simulink model "house_heat_model"  (R2017a)
settings: Solver=ode3  StartTime=0.0  StopTime=1*7*24*3600  FixedStep=dt  RelTol=1e-3  AbsTol=1e-6
model workspace (MATLAB code in the model file):
  | % load initial conditions and physical properties from file
  | 
  | house_heat_model_init
values from neighbouring files (symbols this model uses):
  c_a = simdata.Simulation.Material.c_a.value    [house_heat_model_init.m]
  c_floor = simdata.Simulation.Material.c_floor.value    [house_heat_model_init.m]
  c_s = simdata.Simulation.Material.c_s.value    [house_heat_model_init.m]
  c_water = simdata.Simulation.Material.c_water.value    [house_heat_model_init.m]
  dt = simdata.Simulation.dt.value    [house_heat_model_init.m]
  dT_histerezis = simdata.Simulation.Heat.dT_histerizes.value    [house_heat_model_init.m]
  M_air = (lenHouse*widHouse*htHouse+tan(pitRoof)*widHouse*lenHouse)*densAir    [house_heat_model_init.m]
  M_floor = floorArea*L_floor*densConcrete*heatedPct    [house_heat_model_init.m]
  Mdot = simdata.Simulation.Heat.M_dot.value    [house_heat_model_init.m]
  R_floor = L_floor/(k_floor*floorArea)    [house_heat_model_init.m]
  R_house = R_wall*R_window/(R_wall + R_window)    [house_heat_model_init.m]
  THeater = simdata.Simulation.Heat.T_Heater.value    [house_heat_model_init.m]
  TinIC = simdata.Simulation.Heat.T_IN_ini.value    [house_heat_model_init.m]
libraries: neural x15, dspswit3 x1, simulink x1, powerlib_meascontrol x1
settings Model: ExtModeTrigMode=oneshot  ExtModeArmWhenConnect=off  ExtModeAutoUpdateStatusClock=off  Creator=The MathWorks Inc.  LastModifiedBy=szabo
settings DataIOCC: Decimation=5  ExternalInput=[]  InitialState=[]  SaveFormat=Array  SaveOutput=off  SignalLogging=off  SaveTime=off  SignalLoggingName=sldemo_househeat_output
settings OptimizationCC: BlockReduction=off  BooleanDataType=off  ExpressionDepthLimit=2147483647  InitFltsAndDblsToZero=on  LifeSpan=inf  BufferReusableBoundary=off
settings DebuggingCC: SaveWithParameterizedLinksMsg=none  UnderspecifiedInitializationDetection=Classic  MergeDetectMultiDrivingBlocksExec=none  SignalResolutionControl=TryResolveAllWithWarning  MultiTaskDSMMsg=warning  MultiTaskCondExecSysMsg=none  IntegerOverflowMsg=none  FcnCallInpInsideContextMsg=warning  BusObjectLabelMismatch=none  StateNameClashWarn=warning  SFUnexpectedBacktrackingDiag=warning  SFNoUnconditionalDefaultTransitionDiag=warning  SFExecutionAtInitializationDiag=none  IntegerSaturationMsg=none
settings HardwareCC: ProdBitPerPointer=32  ProdBitPerSizeT=32  ProdBitPerPtrDiffT=32  ProdLargestAtomicFloat=None  ProdIntDivRoundTo=Undefined  ProdEndianess=Unspecified  ProdWordSize=32  ProdHWDeviceType=32-bit Generic  TargetUnknown=on
settings ModelReferenceCC: PropagateSignalLabelsOutOfModel=off
settings GRTTargetCC: TargetFcnLib=ansi_tfl_tmw.mat  TargetLangStandard=C89/C90 (ANSI)  GeneratePreprocessorConditionals=Disable all  CombineOutputUpdateFcns=off  GRTInterface=on
settings ConfigComp: CovMetricSettings=dw  CovHtmlReporting=on  CovSaveCumulativeToWorkspaceVar=on  CovSaveSingleToWorkspaceVar=on  CovExternalEMLEnable=off  CovSFcnEnable=off

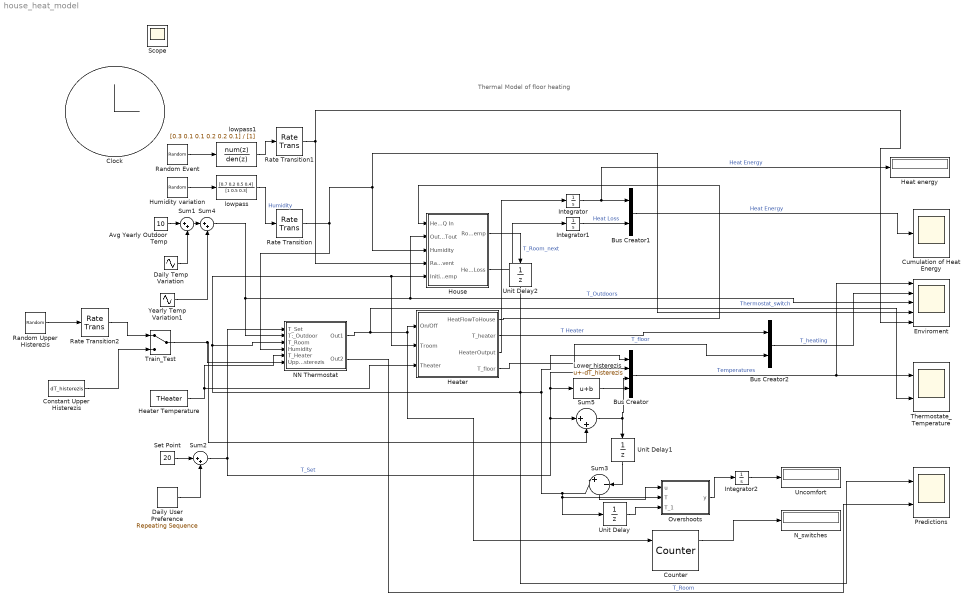
== system house_heat_model ==
  note: Thermal Model of floor heating
  Avg Yearly Outdoor Temp : Constant  Value=10
  Bus Creator : BusCreator  Inputs=4
  Bus Creator1 : BusCreator  Inputs=2
  Bus Creator2 : BusCreator  Inputs=2
  Clock : Clock
  Constant Upper Histerezis : Constant  Value=dT_histerezis  SampleTime=dt
  Counter : dspswit3/Counter  Direction=Up  CountEvent=Rising edge  CounterSize=32 bits  MaxCount=255  InitialCount=0  Output=Count and Hit  HitValue=32  ResetInput=on  SamplesPerFrame=1  Ts=1  CntDtype=double  HitDtype=Logical
  Cumulation of Heat Energy : Scope
  Daily Temp Variation : Sin  Amplitude=5  Frequency=2*pi/(24*3600)  SampleTime=dt
  Daily User Preference : simulink/Sources/Repeating Sequence  rep_seq_t=[0 25199 25200 32399 32400 57599 57600 79199 79200]  rep_seq_y=[-1 -1 1 1 -2 -2 1 1 -1]
  Enviroment : Scope  NumInputPorts=5
  Heat energy : Display
  Heater : Subsystem
      settings: MinAlgLoopOccurrences=on
  Heater Temperature : Constant  Value=THeater
  House : Subsystem
      settings: MinAlgLoopOccurrences=on
      mask Display: image(fullfile(matlabroot,'toolbox','simulink','simdemos','simgeneral','images','HouseHeatHousePix.svg'))
  Humidity variation : RandomNumber  Description=Random events in heat capacity of the room - like window opening, persons in the house, e.t.c  Mean=0.7  Variance=0.05  SampleTime=3600*24
  Integrator : Integrator
  Integrator1 : Integrator
  Integrator2 : Integrator
  Lower histerezis : Bias  Bias=-dT_histerezis
  "NN Thermostat " : Subsystem
      settings: MinAlgLoopOccurrences=on
      mask Display: image(fullfile(matlabroot,'toolbox','simulink','simdemos','simgeneral','images','HouseHeatThermostatPix.svg'))
  N_switches : Display
  Overshoots : MATLAB Function  TreatAsAtomicUnit=on
  Predictions : Scope  NumInputPorts=2
  Random Event : RandomNumber  Mean=1.2  Variance=0.01  SampleTime=3600
  Random Upper Histerezis : UniformRandomNumber  Minimum=0  Maximum=dT_histerezis  SampleTime=3600
  Rate Transition : RateTransition  X0=0.7
  Rate Transition1 : RateTransition  X0=1
  Rate Transition2 : RateTransition  X0=0.25
  Set Point : Constant  Value=20
  Sum{1..2,4..5} (4 alike) : Sum  Inputs=|++  SaturateOnIntegerOverflow=on  InputSameDT=on  OutDataTypeStr=Inherit: Same as first input
  Sum3 : Sum  Inputs=|+||-  SaturateOnIntegerOverflow=on  InputSameDT=on  OutDataTypeStr=Inherit: Same as first input
  Thermostate_Temperature : Scope  NumInputPorts=2
  Train_Test : ManualSwitch
  Uncomfort : Display
  Unit Delay : UnitDelay  InitialCondition=TinIC  SampleTime=-1
  Unit Delay1 : UnitDelay  InitialCondition=TinIC  SampleTime=-1
  Unit Delay2 : UnitDelay  InitialCondition=TinIC  SampleTime=-1
  Yearly Temp Variation1 : Sin  Amplitude=10  Frequency=2*pi/(365*24*3600)  Phase=-3*pi/4  SampleTime=dt
  lowpass : DiscreteFilter  Numerator=[0.7 0.2 0.5 0.4]  Denominator=[1 0.5 0.3]  InitialStates=0.5  SampleTime=3600  a0EqualsOne=on
  lowpass1 : DiscreteFilter  Numerator=[0.3 0.1 0.1 0.2 0.2 0.1]  Denominator=[1]  InitialStates=1  SampleTime=120  a0EqualsOne=on
  Scope : Scope
  wires:
  Integrator/1 -> Heat energy/1, Bus Creator1/1  "Heat Energy"
  Daily Temp Variation/1 -> Sum1/2
  Sum4/1 -> "NN Thermostat "/2(T:_Outdoor), Enviroment/3, House/2(Outdoor Temp Tout)  "T_Outdoors"
  Avg Yearly Outdoor Temp/1 -> Sum1/1
  House/1("Room Temp ") -> Unit Delay2/1  "T_Room_next"
  Heater/1("HeatFlowToHouse ") -> House/1(Heater dQ In)
  Daily User Preference/1 -> Sum2/2
  Set Point/1 -> Sum2/1
  Sum2/1 -> "NN Thermostat "/1(T_Set), Sum5/1, Lower histerezis/1, Bus Creator/2  "T_Set"
  Bus Creator/1 -> Enviroment/1, Thermostate_Temperature/1  "Temperatures"
  Sum5/1 -> Bus Creator/3, Unit Delay1/1
  Random Event/1 -> lowpass1/1
  Heater/3(HeaterOutput) -> Integrator/1
  House/2(Heat Loss) -> Integrator1/1
  Integrator1/1 -> Bus Creator1/2  "Heat Loss"
  Overshoots/1(y) -> Integrator2/1
  Integrator2/1 -> Uncomfort/1
  Counter/1 -> N_switches/1
  Humidity variation/1 -> lowpass/1
  lowpass/1 -> Rate Transition/1  "Humidity"
  lowpass1/1 -> Rate Transition1/1
  "NN Thermostat "/1(Out1) -> Thermostate_Temperature/2, Counter/1, Heater/1(On/Off)  "Thermostat_switch"
  Unit Delay2/1 -> Predictions/1, Heater/2(Troom), House/5("Initial Room Temp "), "NN Thermostat "/3(T_Room), Bus Creator/1, Sum3/1, Overshoots/2(T), Unit Delay/1  "T_Room"
  Sum3/1 -> Overshoots/1(u)
  Unit Delay/1 -> Overshoots/3(T_1)
  Unit Delay1/1 -> Sum3/2
  Lower histerezis/1 -> Bus Creator/4
  "NN Thermostat "/2(Out2) -> Predictions/2
  Rate Transition/1 -> House/3(Humidity), Enviroment/4, "NN Thermostat "/4(Humidity)
  Rate Transition1/1 -> House/4("Random Event "), Enviroment/5
  Heater Temperature/1 -> "NN Thermostat "/5(T_Heater), Heater/3(Theater)
  Sum1/1 -> Sum4/1
  Yearly Temp Variation1/1 -> Sum4/2
  Bus Creator2/1 -> Enviroment/2  "T_heatiing"
  Heater/2("T_heater ") -> Bus Creator2/1  "T Heater"
  Heater/4(T_floor) -> Bus Creator2/2  "T_floor"
  Random Upper Histerezis/1 -> Rate Transition2/1
  Train_Test/1 -> Sum5/2, "NN Thermostat "/6(Upper Histerezis)
  Constant Upper Histerezis/1 -> Train_Test/2
  Rate Transition2/1 -> Train_Test/1
  Bus Creator1/1 -> Cumulation of Heat Energy/1  "Heat Energy"

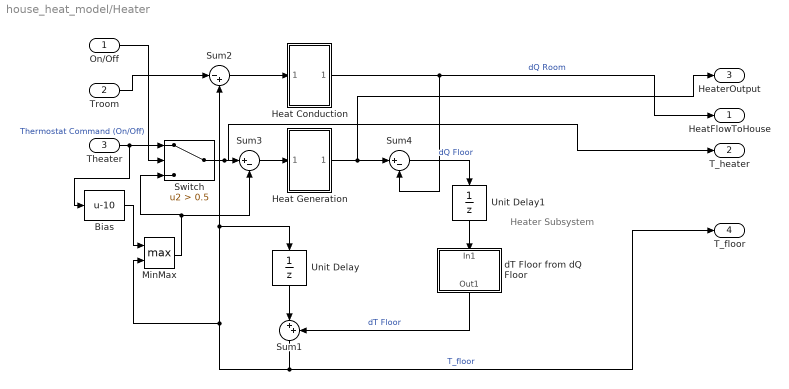
== system house_heat_model/Heater ==
  note: Heater Subsystem
  On/Off : Inport
  Troom : Inport  Port=2
  Theater : Inport  Port=3
  Bias : Bias  Bias=-10
  Heat Generation : Subsystem  Description=assumption: all heater energy is transmitted to the floor and house heating
  Heat Conduction : Subsystem
  MinMax : MinMax  Function=max  Inputs=2
  Sum1 : Sum  Inputs=|++
  Sum2 : Sum  Inputs=|-+
  Sum3 : Sum  Inputs=|+-
  Sum4 : Sum  Inputs=|+-
  Switch : Switch  Criteria=u2 > Threshold  Threshold=0.5
  Unit Delay : UnitDelay  InitialCondition=TinIC  SampleTime=-1
  Unit Delay1 : UnitDelay  InitialCondition=TinIC  SampleTime=-1
  dT Floor from dQ Floor : Subsystem
  "HeatFlowToHouse " : Outport
  "T_heater " : Outport  Port=2
  HeaterOutput : Outport  Port=3
  T_floor : Outport  Port=4
  wires:
  Troom/1 -> Sum2/1
  Sum2/1 -> Heat Conduction/1(In1)
  On/Off/1 -> Switch/2  "Thermostat Command (On/Off)"
  Unit Delay/1 -> Sum1/1
  Sum1/1 -> MinMax/2, Sum2/2, Unit Delay/1, T_floor/1  "T_floor"
  Theater/1 -> Bias/1, Switch/1
  dT Floor from dQ Floor/1(Out1) -> Sum1/2  "dT Floor"
  Heat Conduction/1(Out1) -> "HeatFlowToHouse "/1, Sum4/2  "dQ Room"
  Switch/1 -> "T_heater "/1, Sum3/1
  Sum3/1 -> Heat Generation/1(In1)
  Heat Generation/1(Out1) -> HeaterOutput/1, Sum4/1
  Sum4/1 -> Unit Delay1/1  "dQ Floor"
  Unit Delay1/1 -> dT Floor from dQ Floor/1(In1)
  Bias/1 -> MinMax/1
  MinMax/1 -> Sum3/2, Switch/3

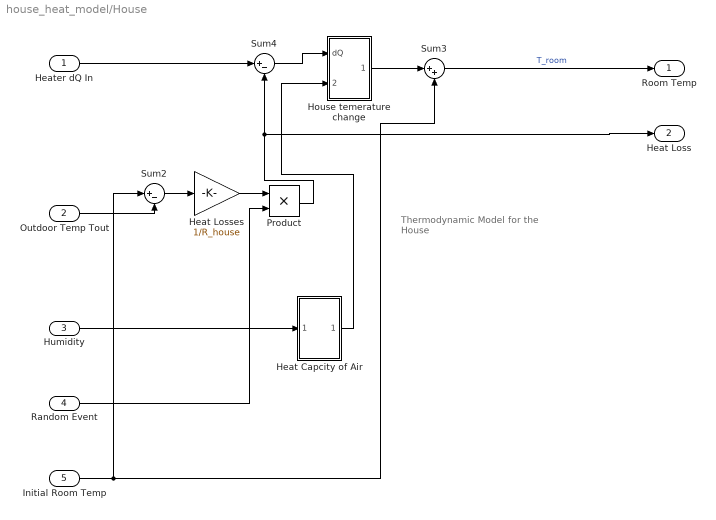
== system house_heat_model/House ==
  note: Thermodynamic Model
      | for the House
  Heater dQ In : Inport
  Outdoor Temp Tout : Inport  Port=2
  Humidity : Inport  Port=3
  "Random Event " : Inport  Port=4
  "Initial Room Temp " : Inport  Port=5
  "Heat Capcity of Air " : Subsystem
  Heat Losses : Gain  Gain=1/R_house  SaturateOnIntegerOverflow=on  OutDataTypeStr=Inherit: Same as input  ParamDataTypeStr=Inherit: Same as input
  House temerature change : Subsystem
  Product : Product
  Sum2 : Sum  Inputs=|+-  SaturateOnIntegerOverflow=on  InputSameDT=on  OutDataTypeStr=Inherit: Same as first input
  Sum3 : Sum  Inputs=|++
  Sum4 : Sum  Inputs=|+-  SaturateOnIntegerOverflow=on  InputSameDT=on  OutDataTypeStr=Inherit: Same as first input
  "Room Temp " : Outport  InitialOutput=0
  Heat Loss : Outport  Port=2  InitialOutput=0
  wires:
  Outdoor Temp Tout/1 -> Sum2/2
  Sum2/1 -> Heat Losses/1
  Sum3/1 -> "Room Temp "/1  "T_room"
  Heater dQ In/1 -> Sum4/1
  House temerature change/1(Out1) -> Sum3/1
  Sum4/1 -> House temerature change/1(dQ)
  Humidity/1 -> "Heat Capcity of Air "/1(In1)
  "Heat Capcity of Air "/1(Out1) -> House temerature change/2(Heat Capacity)
  "Random Event "/1 -> Product/2
  Heat Losses/1 -> Product/1
  Product/1 -> Heat Loss/1, Sum4/2
  "Initial Room Temp "/1 -> Sum2/1, Sum3/2

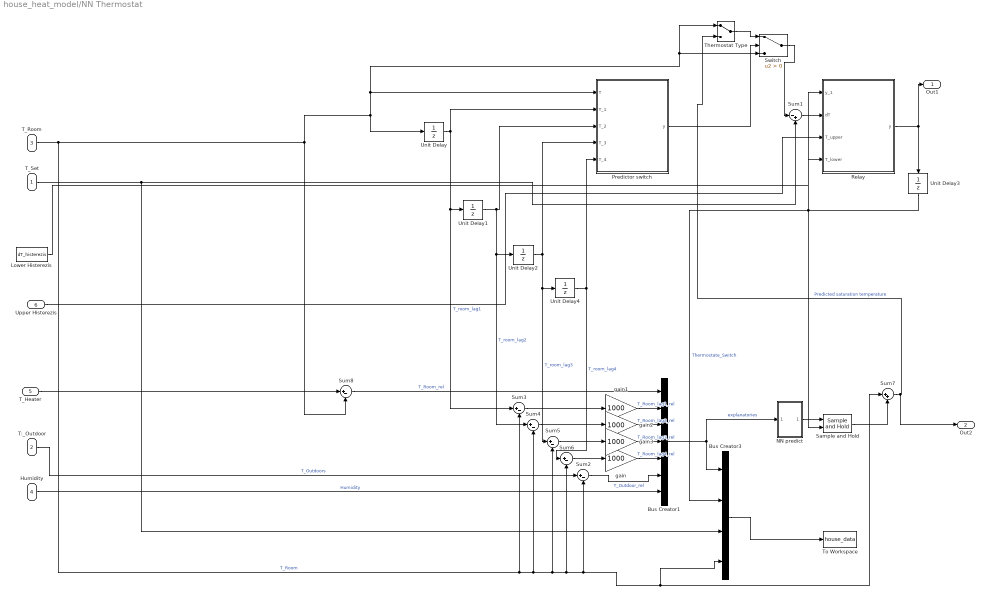
== system house_heat_model/NN Thermostat  ==
  T_Set : Inport
  T:_Outdoor : Inport  Port=2
  T_Room : Inport  Port=3
  Humidity : Inport  Port=4
  T_Heater : Inport  Port=5
  Upper Histerezis : Inport  Port=6
  Bus Creator1 : BusCreator  Inputs=7
  Bus Creator3 : BusCreator  Inputs=4
  Lower Histerezis : Constant  Value=dT_histerezis
  NN predict : Subsystem
  Predictor switch : MATLAB Function  TreatAsAtomicUnit=on
  Relay : MATLAB Function  TreatAsAtomicUnit=on
  Sample and Hold : powerlib_meascontrol/Additional Components/Sample and Hold  ic=0  Ts=dt
      settings: SourceProductName=Simscape Power Systems  SourceProductBaseCode=PS
  Sum1 : Sum  Inputs=|-+  SaturateOnIntegerOverflow=on  InputSameDT=on  OutDataTypeStr=Inherit: Same as first input
  Sum{2..6,8} (6 alike) : Sum  Inputs=|+-  SaturateOnIntegerOverflow=on  InputSameDT=on  OutDataTypeStr=Inherit: Same as first input
  Sum7 : Sum  Inputs=|++  SaturateOnIntegerOverflow=on  InputSameDT=on  OutDataTypeStr=Inherit: Same as first input
  Switch : Switch  Criteria=u2 > Threshold
  Thermostat Type : ManualSwitch  Description=|
      | Turn on/off smart thermostat
      | Off: Up
      | On: Down
  To Workspace : ToWorkspace  VariableName=house_data  SaveFormat=Timeseries  SampleTime=-1
  Unit Delay{,1..2,4} (4 alike) : UnitDelay  InitialCondition=TinIC  SampleTime=-1
  Unit Delay3 : UnitDelay  SampleTime=-1
  gain{,1..3} (4 alike) : Gain  Gain=1000
  Out1 : Outport
  Out2 : Outport  Port=2
  wires:
  Unit Delay/1 -> Predictor switch/2(T_1), Sum3/1, Unit Delay1/1  "T_room_lag1"
  Relay/1(y) -> Out1/1, Unit Delay3/1
  Switch/1 -> Sum1/1
  Unit Delay1/1 -> Predictor switch/3(T_2), Unit Delay2/1, Sum4/1  "T_room_lag2"
  Predictor switch/1(y) -> Switch/2
  Unit Delay2/1 -> Unit Delay4/1, Sum5/1, Predictor switch/4(T_3)  "T_room_lag3"
  Unit Delay3/1 -> Relay/1(y_1), Sample and Hold/2, Bus Creator3/2  "Thermostate_Switch"
  Thermostat Type/1 -> Switch/1
  T_Room/1 -> Sum8/2, Predictor switch/1(T), Thermostat Type/1, Switch/3, Unit Delay/1, Sum7/1, Bus Creator3/4, Sum2/2, Sum6/2, Sum5/2, Sum4/2, Sum3/2  "T_Room"
  Bus Creator3/1 -> To Workspace/1
  NN predict/1(Out1) -> Sample and Hold/1
  Sum3/1 -> gain1/1
  Sum4/1 -> gain2/1
  Sum5/1 -> gain3/1
  Sum6/1 -> gain/1
  Humidity/1 -> Bus Creator1/7  "Humidity"
  Bus Creator1/1 -> NN predict/1(In1), Bus Creator3/1  "explanatories"
  Sample and Hold/1 -> Sum7/2
  T_Set/1 -> Bus Creator3/3, Sum1/2
  Sum7/1 -> Out2/1, Thermostat Type/2  "Predicted saturation temperature"
  Sum2/1 -> Bus Creator1/6  "T_Outdoor_rel"
  Unit Delay4/1 -> Predictor switch/5(T_4), Sum6/1  "T_room_lag4"
  T:_Outdoor/1 -> Sum2/1  "T_Outdoors"
  T_Heater/1 -> Sum8/1
  Sum8/1 -> Bus Creator1/1  "T_Room_rel"
  Lower Histerezis/1 -> Relay/4(T_lower)
  Upper Histerezis/1 -> Relay/3(T_upper)
  gain1/1 -> Bus Creator1/2  "T_Room_lag1_rel"
  gain2/1 -> Bus Creator1/3  "T_Room_lag2_rel"
  gain3/1 -> Bus Creator1/4  "T_Room_lag3_rel"
  gain/1 -> Bus Creator1/5  "T_Room_lag4_rel"
  Sum1/1 -> Relay/2(dT)

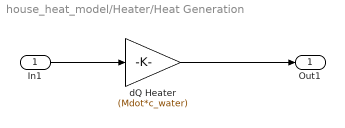
== system house_heat_model/Heater/Heat Generation ==
  In1 : Inport
  dQ Heater : Gain  Gain=(Mdot*c_water)
  Out1 : Outport
  wires:
  In1/1 -> dQ Heater/1
  dQ Heater/1 -> Out1/1

== system house_heat_model/Heater/Heat Conduction ==
  In1 : Inport
  Heat conduction : Gain  Gain=1/R_floor
  Out1 : Outport
  wires:
  In1/1 -> Heat conduction/1
  Heat conduction/1 -> Out1/1

== system house_heat_model/Heater/dT Floor from dQ Floor ==
  In1 : Inport
  Floor Incapacity : Gain  Gain=dt/(M_floor*c_floor)
  Out1 : Outport
  wires:
  In1/1 -> Floor Incapacity/1
  Floor Incapacity/1 -> Out1/1  "dT Floor"

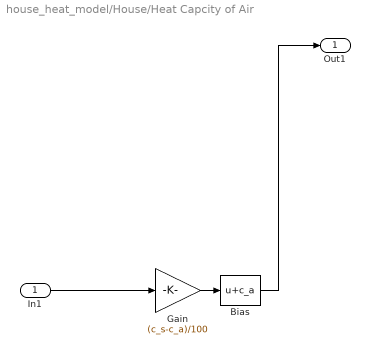
== system house_heat_model/House/Heat Capcity of Air  ==
  In1 : Inport
  Bias : Bias  Bias=c_a
  Gain : Gain  Gain=(c_s-c_a)/100  SaturateOnIntegerOverflow=on  OutDataTypeStr=Inherit: Same as input  ParamDataTypeStr=Inherit: Same as input
  Out1 : Outport
  wires:
  In1/1 -> Gain/1
  Bias/1 -> Out1/1
  Gain/1 -> Bias/1

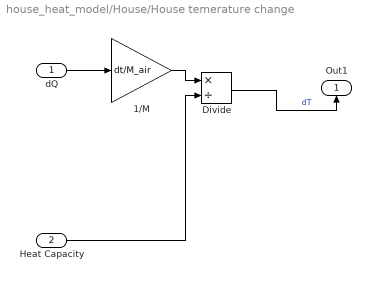
== system house_heat_model/House/House temerature change ==
  dQ : Inport
  Heat Capacity : Inport  Port=2
  1/M : Gain  Gain=dt/M_air  SaturateOnIntegerOverflow=on  OutDataTypeStr=Inherit: Same as input  ParamDataTypeStr=Inherit: Same as input
  Divide : Product  Inputs=*/
  Out1 : Outport
  wires:
  1/M/1 -> Divide/1
  dQ/1 -> 1/M/1
  Divide/1 -> Out1/1  "dT"
  Heat Capacity/1 -> Divide/2

== system house_heat_model/NN Thermostat /NN predict ==
  In1 : Inport
  Function Fitting Neural Network1 : Subsystem
      mask help: Function Fitting Neural Network
      mask Display: e = 0.06;c1 = [120 150 230]/255;c2 = ([120 150 230]+0)/383;c3 = ([120 150 230]+128)/383;patch([0 1 1 0],[0 0 1 1],c1);patch([0 1 1 1-e 1-e 0+e],[0 0 1 1-e 0+e 0+e],c2);patch([0 0 1 1-e 0+e 0+e],[0 1 1 1-e 1-e 0+e],c3);plot([0 1 1 0 0],[0 0 1 1 0]);fprintf('NNET');port_label('input',1,' Input');port_label('output',1,'Output ');
  Out1 : Outport
  wires:
  In1/1 -> Function Fitting Neural Network1/1(Input)
  Function Fitting Neural Network1/1(Output) -> Out1/1

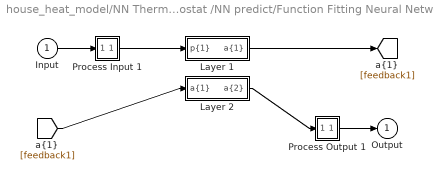
== system house_heat_model/NN Thermostat /NN predict/Function Fitting Neural Network1 ==
  Input : Inport  PortDimensions=7  SampleTime=10
      mask Display: e = 0.06;c1 = [120 230 180]/255;c2 = ([120 230 180]+0)/(256+128);c3 = ([120 230 180]+128)/(256+128);patch([0 1 1 0],[0 0 1 1],c1);patch([0 1 1 1-e 1-e 0+e],[0 0 1 1-e 0+e 0+e],c2);patch([0 0 1 1-e 0+e 0+e],[0 1 1 1-e 1-e 0+e],c3);plot([0 1 1 0 0],[0 0 1 1 0]);
  Layer 1 : Subsystem
      mask Display: e = 0.06;c1 = [120 150 230]/255;c2 = ([120 150 230]+0)/383;c3 = ([120 150 230]+128)/383;patch([0 1 1 0],[0 0 1 1],c1);patch([0 1 1 1-e 1-e 0+e],[0 0 1 1-e 0+e 0+e],c2);patch([0 0 1 1-e 0+e 0+e],[0 1 1 1-e 1-e 0+e],c3);plot([0 1 1 0 0],[0 0 1 1 0]);
  Layer 2 : Subsystem
      mask Display: e = 0.06;c1 = [120 150 230]/255;c2 = ([120 150 230]+0)/383;c3 = ([120 150 230]+128)/383;patch([0 1 1 0],[0 0 1 1],c1);patch([0 1 1 1-e 1-e 0+e],[0 0 1 1-e 0+e 0+e],c2);patch([0 0 1 1-e 0+e 0+e],[0 1 1 1-e 1-e 0+e],c3);plot([0 1 1 0 0],[0 0 1 1 0]);
  Process Input 1 : Subsystem
      mask Display: e = 0.06;c1 = [120 150 230]/255;c2 = ([120 150 230]+0)/383;c3 = ([120 150 230]+128)/383;patch([0 1 1 0],[0 0 1 1],c1);patch([0 1 1 1-e 1-e 0+e],[0 0 1 1-e 0+e 0+e],c2);patch([0 0 1 1-e 0+e 0+e],[0 1 1 1-e 1-e 0+e],c3);plot([0 1 1 0 0],[0 0 1 1 0]);
  Process Output 1 : Subsystem
      mask Display: e = 0.06;c1 = [120 150 230]/255;c2 = ([120 150 230]+0)/383;c3 = ([120 150 230]+128)/383;patch([0 1 1 0],[0 0 1 1],c1);patch([0 1 1 1-e 1-e 0+e],[0 0 1 1-e 0+e 0+e],c2);patch([0 0 1 1-e 0+e 0+e],[0 1 1 1-e 1-e 0+e],c3);plot([0 1 1 0 0],[0 0 1 1 0]);
  Output : Outport  InitialOutput=0
      mask Display: e = 0.06;c1 = [120 230 180]/255;c2 = ([120 230 180]+0)/(256+128);c3 = ([120 230 180]+128)/(256+128);patch([0 1 1 0],[0 0 1 1],c1);patch([0 1 1 1-e 1-e 0+e],[0 0 1 1-e 0+e 0+e],c2);patch([0 0 1 1-e 0+e 0+e],[0 1 1 1-e 1-e 0+e],c3);plot([0 1 1 0 0],[0 0 1 1 0]);
  wires:
  Input/1 -> Process Input 1/1(x)
  Process Output 1/1(y) -> Output/1
  Process Input 1/1(p) -> Layer 1/1("p{1}")
  Layer 1/1("a{1}") -> [feedback1]
  [feedback1] -> Layer 2/1("a{1} ")
  Layer 2/1("a{2}") -> Process Output 1/1(a)

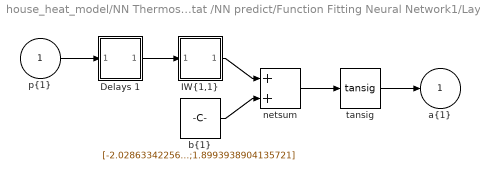
== system house_heat_model/NN Thermostat /NN predict/Function Fitting Neural Network1/Layer 1 ==
  "p{1}" : Inport  PortDimensions=7  SampleTime=10
      mask Display: e = 0.06;c1 = [120 230 180]/255;c2 = ([120 230 180]+0)/(256+128);c3 = ([120 230 180]+128)/(256+128);patch([0 1 1 0],[0 0 1 1],c1);patch([0 1 1 1-e 1-e 0+e],[0 0 1 1-e 0+e 0+e],c2);patch([0 0 1 1-e 0+e 0+e],[0 1 1 1-e 1-e 0+e],c3);plot([0 1 1 0 0],[0 0 1 1 0]);
  Delays 1 : Subsystem
      mask Display: e = 0.06;c1 = [120 150 230]/255;c2 = ([120 150 230]+0)/383;c3 = ([120 150 230]+128)/383;patch([0 1 1 0],[0 0 1 1],c1);patch([0 1 1 1-e 1-e 0+e],[0 0 1 1-e 0+e 0+e],c2);patch([0 0 1 1-e 0+e 0+e],[0 1 1 1-e 1-e 0+e],c3);plot([0 1 1 0 0],[0 0 1 1 0]);disp('0');
  "IW{1,1}" : Subsystem
      mask Display: e = 0.06;c1 = [120 150 230]/255;c2 = ([120 150 230]+0)/383;c3 = ([120 150 230]+128)/383;patch([0 1 1 0],[0 0 1 1],c1);patch([0 1 1 1-e 1-e 0+e],[0 0 1 1-e 0+e 0+e],c2);patch([0 0 1 1-e 0+e 0+e],[0 1 1 1-e 1-e 0+e],c3);plot([0 1 1 0 0],[0 0 1 1 0]);disp('W');
  "b{1}" : Constant  Value=[-2.0286334225674025;-1.4486400293574533;1.0412205681455498;-0.21683670702065122;-0.19472794721376627;-0.15744678412465296;-0.6019783225289782;0.33692757286718333;1.6293452403211961;1.8993938904135721]
      mask Display: e = 0.06;c1 = [120 150 230]/255;c2 = ([120 150 230]+0)/383;c3 = ([120 150 230]+128)/383;patch([0 1 1 0],[0 0 1 1],c1);patch([0 1 1 1-e 1-e 0+e],[0 0 1 1-e 0+e 0+e],c2);patch([0 0 1 1-e 0+e 0+e],[0 1 1 1-e 1-e 0+e],c3);plot([0 1 1 0 0],[0 0 1 1 0]);disp('b');
  netsum : Sum  Inputs=2  SaturateOnIntegerOverflow=on  InputSameDT=on  OutDataTypeStr=Inherit: Same as first input
      mask Display: e = 0.06;c1 = [120 150 230]/255;c2 = ([120 150 230]+0)/383;c3 = ([120 150 230]+128)/383;patch([0 1 1 0],[0 0 1 1],c1);patch([0 1 1 1-e 1-e 0+e],[0 0 1 1-e 0+e 0+e],c2);patch([0 0 1 1-e 0+e 0+e],[0 1 1 1-e 1-e 0+e],c3);plot([0 1 1 0 0],[0 0 1 1 0]);disp('+');
  tansig : neural/Transfer Functions/tansig
  "a{1}" : Outport  InitialOutput=[0;0;0;0;0;0;0;0;0;0]
      mask Display: e = 0.06;c1 = [120 230 180]/255;c2 = ([120 230 180]+0)/(256+128);c3 = ([120 230 180]+128)/(256+128);patch([0 1 1 0],[0 0 1 1],c1);patch([0 1 1 1-e 1-e 0+e],[0 0 1 1-e 0+e 0+e],c2);patch([0 0 1 1-e 0+e 0+e],[0 1 1 1-e 1-e 0+e],c3);plot([0 1 1 0 0],[0 0 1 1 0]);
  wires:
  "p{1}"/1 -> Delays 1/1("p{1}")
  Delays 1/1("pd{1,1}") -> "IW{1,1}"/1("pd{1,1}")
  "IW{1,1}"/1("iz{1,1}") -> netsum/1
  "b{1}"/1 -> netsum/2
  netsum/1 -> tansig/1
  tansig/1 -> "a{1}"/1

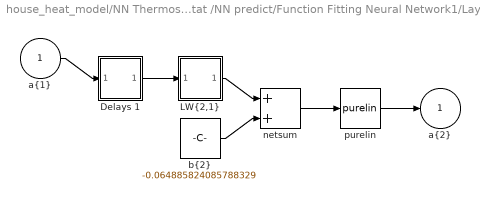
== system house_heat_model/NN Thermostat /NN predict/Function Fitting Neural Network1/Layer 2 ==
  "a{1} " : Inport  PortDimensions=10  SampleTime=10
      mask Display: e = 0.06;c1 = [120 230 180]/255;c2 = ([120 230 180]+0)/(256+128);c3 = ([120 230 180]+128)/(256+128);patch([0 1 1 0],[0 0 1 1],c1);patch([0 1 1 1-e 1-e 0+e],[0 0 1 1-e 0+e 0+e],c2);patch([0 0 1 1-e 0+e 0+e],[0 1 1 1-e 1-e 0+e],c3);plot([0 1 1 0 0],[0 0 1 1 0]);
  Delays 1 : Subsystem
      mask Display: e = 0.06;c1 = [120 150 230]/255;c2 = ([120 150 230]+0)/383;c3 = ([120 150 230]+128)/383;patch([0 1 1 0],[0 0 1 1],c1);patch([0 1 1 1-e 1-e 0+e],[0 0 1 1-e 0+e 0+e],c2);patch([0 0 1 1-e 0+e 0+e],[0 1 1 1-e 1-e 0+e],c3);plot([0 1 1 0 0],[0 0 1 1 0]);disp('0');
  "LW{2,1}" : Subsystem
      mask Display: e = 0.06;c1 = [120 150 230]/255;c2 = ([120 150 230]+0)/383;c3 = ([120 150 230]+128)/383;patch([0 1 1 0],[0 0 1 1],c1);patch([0 1 1 1-e 1-e 0+e],[0 0 1 1-e 0+e 0+e],c2);patch([0 0 1 1-e 0+e 0+e],[0 1 1 1-e 1-e 0+e],c3);plot([0 1 1 0 0],[0 0 1 1 0]);disp('W');
  "b{2}" : Constant  Value=-0.064885824085788329
      mask Display: e = 0.06;c1 = [120 150 230]/255;c2 = ([120 150 230]+0)/383;c3 = ([120 150 230]+128)/383;patch([0 1 1 0],[0 0 1 1],c1);patch([0 1 1 1-e 1-e 0+e],[0 0 1 1-e 0+e 0+e],c2);patch([0 0 1 1-e 0+e 0+e],[0 1 1 1-e 1-e 0+e],c3);plot([0 1 1 0 0],[0 0 1 1 0]);disp('b');
  netsum : Sum  Inputs=2  SaturateOnIntegerOverflow=on  InputSameDT=on  OutDataTypeStr=Inherit: Same as first input
      mask Display: e = 0.06;c1 = [120 150 230]/255;c2 = ([120 150 230]+0)/383;c3 = ([120 150 230]+128)/383;patch([0 1 1 0],[0 0 1 1],c1);patch([0 1 1 1-e 1-e 0+e],[0 0 1 1-e 0+e 0+e],c2);patch([0 0 1 1-e 0+e 0+e],[0 1 1 1-e 1-e 0+e],c3);plot([0 1 1 0 0],[0 0 1 1 0]);disp('+');
  purelin : neural/Transfer Functions/purelin
  "a{2}" : Outport  InitialOutput=0
      mask Display: e = 0.06;c1 = [120 230 180]/255;c2 = ([120 230 180]+0)/(256+128);c3 = ([120 230 180]+128)/(256+128);patch([0 1 1 0],[0 0 1 1],c1);patch([0 1 1 1-e 1-e 0+e],[0 0 1 1-e 0+e 0+e],c2);patch([0 0 1 1-e 0+e 0+e],[0 1 1 1-e 1-e 0+e],c3);plot([0 1 1 0 0],[0 0 1 1 0]);
  wires:
  "a{1} "/1 -> Delays 1/1("p{2}")
  Delays 1/1("pd{2,1}") -> "LW{2,1}"/1("ad{2,1}")
  "LW{2,1}"/1("lz{2,1}") -> netsum/1
  "b{2}"/1 -> netsum/2
  netsum/1 -> purelin/1
  purelin/1 -> "a{2}"/1

== system house_heat_model/NN Thermostat /NN predict/Function Fitting Neural Network1/Process Input 1 ==
  x : Inport  PortDimensions=7  SampleTime=10
      mask Display: e = 0.06;c1 = [120 230 180]/255;c2 = ([120 230 180]+0)/(256+128);c3 = ([120 230 180]+128)/(256+128);patch([0 1 1 0],[0 0 1 1],c1);patch([0 1 1 1-e 1-e 0+e],[0 0 1 1-e 0+e 0+e],c2);patch([0 0 1 1-e 0+e 0+e],[0 1 1 1-e 1-e 0+e],c3);plot([0 1 1 0 0],[0 0 1 1 0]);
  mapminmax : neural/Processing Functions/mapminmax  xmin=[18.471707921307942;-48.861334729174644;-97.621256457170347;-146.23814290682091;-194.66612173058451;-24.031734702265108;0.28463048034998678]  xmax=[21.499974565246148;-0.46489295406004771;-0.92899992107220442;-1.3923231944659165;-1.8548650562877356;-10.857696363779318;1.1742339478717254]  ymin=-1  ymax=1
  p : Outport  PortDimensions=7  SampleTime=10
      mask Display: e = 0.06;c1 = [120 230 180]/255;c2 = ([120 230 180]+0)/(256+128);c3 = ([120 230 180]+128)/(256+128);patch([0 1 1 0],[0 0 1 1],c1);patch([0 1 1 1-e 1-e 0+e],[0 0 1 1-e 0+e 0+e],c2);patch([0 0 1 1-e 0+e 0+e],[0 1 1 1-e 1-e 0+e],c3);plot([0 1 1 0 0],[0 0 1 1 0]);
  wires:
  x/1 -> mapminmax/1
  mapminmax/1 -> p/1

== system house_heat_model/NN Thermostat /NN predict/Function Fitting Neural Network1/Process Output 1 ==
  a : Inport  PortDimensions=1  SampleTime=10
      mask Display: e = 0.06;c1 = [120 230 180]/255;c2 = ([120 230 180]+0)/(256+128);c3 = ([120 230 180]+128)/(256+128);patch([0 1 1 0],[0 0 1 1],c1);patch([0 1 1 1-e 1-e 0+e],[0 0 1 1-e 0+e 0+e],c2);patch([0 0 1 1-e 0+e 0+e],[0 1 1 1-e 1-e 0+e],c3);plot([0 1 1 0 0],[0 0 1 1 0]);
  mapminmax_reverse : neural/Processing Functions/mapminmax_reverse  xmin=0.00046568124321311188  xmax=1.7821580572261553  ymin=-1  ymax=1
  y : Outport  PortDimensions=1  SampleTime=10
      mask Display: e = 0.06;c1 = [120 230 180]/255;c2 = ([120 230 180]+0)/(256+128);c3 = ([120 230 180]+128)/(256+128);patch([0 1 1 0],[0 0 1 1],c1);patch([0 1 1 1-e 1-e 0+e],[0 0 1 1-e 0+e 0+e],c2);patch([0 0 1 1-e 0+e 0+e],[0 1 1 1-e 1-e 0+e],c3);plot([0 1 1 0 0],[0 0 1 1 0]);
  wires:
  a/1 -> mapminmax_reverse/1
  mapminmax_reverse/1 -> y/1

== system house_heat_model/NN Thermostat /NN predict/Function Fitting Neural Network1/Layer 1/Delays 1 ==
  "p{1}" : Inport  PortDimensions=7  SampleTime=10
      mask Display: e = 0.06;c1 = [120 230 180]/255;c2 = ([120 230 180]+0)/(256+128);c3 = ([120 230 180]+128)/(256+128);patch([0 1 1 0],[0 0 1 1],c1);patch([0 1 1 1-e 1-e 0+e],[0 0 1 1-e 0+e 0+e],c2);patch([0 0 1 1-e 0+e 0+e],[0 1 1 1-e 1-e 0+e],c3);plot([0 1 1 0 0],[0 0 1 1 0]);
  mux : Mux  Inputs=1
      mask Display: e = 0.06;c1 = [120 150 230]/255;c2 = ([120 150 230]+0)/383;c3 = ([120 150 230]+128)/383;patch([0 1 1 0],[0 0 1 1],c1);patch([0 1 1 1-e 1-e 0+e],[0 0 1 1-e 0+e 0+e],c2);patch([0 0 1 1-e 0+e 0+e],[0 1 1 1-e 1-e 0+e],c3);plot([0 1 1 0 0],[0 0 1 1 0]);disp('Mux')
  "pd{1,1}" : Outport
      mask Display: e = 0.06;c1 = [120 230 180]/255;c2 = ([120 230 180]+0)/(256+128);c3 = ([120 230 180]+128)/(256+128);patch([0 1 1 0],[0 0 1 1],c1);patch([0 1 1 1-e 1-e 0+e],[0 0 1 1-e 0+e 0+e],c2);patch([0 0 1 1-e 0+e 0+e],[0 1 1 1-e 1-e 0+e],c3);plot([0 1 1 0 0],[0 0 1 1 0]);
  wires:
  "p{1}"/1 -> mux/1
  mux/1 -> "pd{1,1}"/1

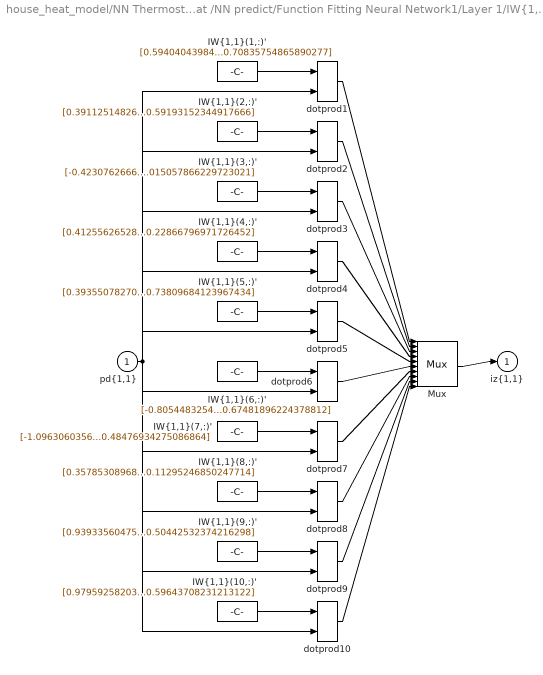
== system house_heat_model/NN Thermostat /NN predict/Function Fitting Neural Network1/Layer 1/IW{1,1} ==
  "pd{1,1}" : Inport  PortDimensions=7  SampleTime=10
      mask Display: e = 0.06;c1 = [120 230 180]/255;c2 = ([120 230 180]+0)/(256+128);c3 = ([120 230 180]+128)/(256+128);patch([0 1 1 0],[0 0 1 1],c1);patch([0 1 1 1-e 1-e 0+e],[0 0 1 1-e 0+e 0+e],c2);patch([0 0 1 1-e 0+e 0+e],[0 1 1 1-e 1-e 0+e],c3);plot([0 1 1 0 0],[0 0 1 1 0]);
  "IW{1,1}(1,:)'" : Constant  Value=[0.59404043984043264;-1.1003291766529382;0.43904004160616333;0.59862140949124887;-0.21632364014253425;-0.74454594146497333;0.70835754865890277]
      mask Display: e = 0.06;c1 = [120 150 230]/255;c2 = ([120 150 230]+0)/383;c3 = ([120 150 230]+128)/383;patch([0 1 1 0],[0 0 1 1],c1);patch([0 1 1 1-e 1-e 0+e],[0 0 1 1-e 0+e 0+e],c2);patch([0 0 1 1-e 0+e 0+e],[0 1 1 1-e 1-e 0+e],c3);plot([0 1 1 0 0],[0 0 1 1 0]);disp('Weights');
  "IW{1,1}(10,:)'" : Constant  Value=[0.97959258203271249;0.91999223565181143;-0.65113965867611268;-0.92348934903008351;0.52192515519142624;-0.44380734871779914;-0.59643708231213122]
      mask Display: e = 0.06;c1 = [120 150 230]/255;c2 = ([120 150 230]+0)/383;c3 = ([120 150 230]+128)/383;patch([0 1 1 0],[0 0 1 1],c1);patch([0 1 1 1-e 1-e 0+e],[0 0 1 1-e 0+e 0+e],c2);patch([0 0 1 1-e 0+e 0+e],[0 1 1 1-e 1-e 0+e],c3);plot([0 1 1 0 0],[0 0 1 1 0]);disp('Weights');
  "IW{1,1}(2,:)'" : Constant  Value=[0.39112514826830741;0.89551385792533955;-0.98741253551403629;-0.99329317953234775;-0.27469918480348804;0.2026601980782545;-0.59193152344917666]
      mask Display: e = 0.06;c1 = [120 150 230]/255;c2 = ([120 150 230]+0)/383;c3 = ([120 150 230]+128)/383;patch([0 1 1 0],[0 0 1 1],c1);patch([0 1 1 1-e 1-e 0+e],[0 0 1 1-e 0+e 0+e],c2);patch([0 0 1 1-e 0+e 0+e],[0 1 1 1-e 1-e 0+e],c3);plot([0 1 1 0 0],[0 0 1 1 0]);disp('Weights');
  "IW{1,1}(3,:)'" : Constant  Value=[-0.42307626660140019;0.98368546246326016;0.70825853997448562;-0.71257444565578765;0.49036557648571133;0.54720614452339766;0.015057866229723021]
      mask Display: e = 0.06;c1 = [120 150 230]/255;c2 = ([120 150 230]+0)/383;c3 = ([120 150 230]+128)/383;patch([0 1 1 0],[0 0 1 1],c1);patch([0 1 1 1-e 1-e 0+e],[0 0 1 1-e 0+e 0+e],c2);patch([0 0 1 1-e 0+e 0+e],[0 1 1 1-e 1-e 0+e],c3);plot([0 1 1 0 0],[0 0 1 1 0]);disp('Weights');
  "IW{1,1}(4,:)'" : Constant  Value=[0.41255626528578004;0.086286222305269972;0.9953349420006038;-0.95946818733913486;0.57279696068862473;-0.14934312136702033;-0.22866796971726452]
      mask Display: e = 0.06;c1 = [120 150 230]/255;c2 = ([120 150 230]+0)/383;c3 = ([120 150 230]+128)/383;patch([0 1 1 0],[0 0 1 1],c1);patch([0 1 1 1-e 1-e 0+e],[0 0 1 1-e 0+e 0+e],c2);patch([0 0 1 1-e 0+e 0+e],[0 1 1 1-e 1-e 0+e],c3);plot([0 1 1 0 0],[0 0 1 1 0]);disp('Weights');
  "IW{1,1}(5,:)'" : Constant  Value=[0.39355078270908928;0.69726249563590748;0.44106077327171156;-0.89477439624527355;-0.64835527416620842;-0.69152226632227698;0.73809684123967434]
      mask Display: e = 0.06;c1 = [120 150 230]/255;c2 = ([120 150 230]+0)/383;c3 = ([120 150 230]+128)/383;patch([0 1 1 0],[0 0 1 1],c1);patch([0 1 1 1-e 1-e 0+e],[0 0 1 1-e 0+e 0+e],c2);patch([0 0 1 1-e 0+e 0+e],[0 1 1 1-e 1-e 0+e],c3);plot([0 1 1 0 0],[0 0 1 1 0]);disp('Weights');
  "IW{1,1}(6,:)'" : Constant  Value=[-0.80544832545231126;-0.57381608146254015;0.88063161396307199;1.0343770335625775;0.23089434869096556;-0.3135925422653198;0.67481896224378812]
      mask Display: e = 0.06;c1 = [120 150 230]/255;c2 = ([120 150 230]+0)/383;c3 = ([120 150 230]+128)/383;patch([0 1 1 0],[0 0 1 1],c1);patch([0 1 1 1-e 1-e 0+e],[0 0 1 1-e 0+e 0+e],c2);patch([0 0 1 1-e 0+e 0+e],[0 1 1 1-e 1-e 0+e],c3);plot([0 1 1 0 0],[0 0 1 1 0]);disp('Weights');
  "IW{1,1}(7,:)'" : Constant  Value=[-1.0963060356431378;-0.25560362674956549;0.76674162166900828;0.60838616294281966;-0.21587841826507459;0.95094445594872701;0.48476934275086864]
      mask Display: e = 0.06;c1 = [120 150 230]/255;c2 = ([120 150 230]+0)/383;c3 = ([120 150 230]+128)/383;patch([0 1 1 0],[0 0 1 1],c1);patch([0 1 1 1-e 1-e 0+e],[0 0 1 1-e 0+e 0+e],c2);patch([0 0 1 1-e 0+e 0+e],[0 1 1 1-e 1-e 0+e],c3);plot([0 1 1 0 0],[0 0 1 1 0]);disp('Weights');
  "IW{1,1}(8,:)'" : Constant  Value=[0.35785308968660717;1.4506898829064991;-0.1694559310799032;-0.40160190065356244;0.59241696342103667;-0.43516816669783709;-0.11295246850247714]
      mask Display: e = 0.06;c1 = [120 150 230]/255;c2 = ([120 150 230]+0)/383;c3 = ([120 150 230]+128)/383;patch([0 1 1 0],[0 0 1 1],c1);patch([0 1 1 1-e 1-e 0+e],[0 0 1 1-e 0+e 0+e],c2);patch([0 0 1 1-e 0+e 0+e],[0 1 1 1-e 1-e 0+e],c3);plot([0 1 1 0 0],[0 0 1 1 0]);disp('Weights');
  "IW{1,1}(9,:)'" : Constant  Value=[0.93933560475185685;0.73964479352626533;0.41845337357163198;1.1042509198673196;0.5187505276227139;0.091467070137879719;-0.50442532374216298]
      mask Display: e = 0.06;c1 = [120 150 230]/255;c2 = ([120 150 230]+0)/383;c3 = ([120 150 230]+128)/383;patch([0 1 1 0],[0 0 1 1],c1);patch([0 1 1 1-e 1-e 0+e],[0 0 1 1-e 0+e 0+e],c2);patch([0 0 1 1-e 0+e 0+e],[0 1 1 1-e 1-e 0+e],c3);plot([0 1 1 0 0],[0 0 1 1 0]);disp('Weights');
  Mux : Mux  Inputs=10
      mask Display: e = 0.06;c1 = [120 150 230]/255;c2 = ([120 150 230]+0)/383;c3 = ([120 150 230]+128)/383;patch([0 1 1 0],[0 0 1 1],c1);patch([0 1 1 1-e 1-e 0+e],[0 0 1 1-e 0+e 0+e],c2);patch([0 0 1 1-e 0+e 0+e],[0 1 1 1-e 1-e 0+e],c3);plot([0 1 1 0 0],[0 0 1 1 0]);disp('Mux');
  dotprod{1..10} (10 alike) : neural/Weight Functions/dotprod
  "iz{1,1}" : Outport
      mask Display: e = 0.06;c1 = [120 230 180]/255;c2 = ([120 230 180]+0)/(256+128);c3 = ([120 230 180]+128)/(256+128);patch([0 1 1 0],[0 0 1 1],c1);patch([0 1 1 1-e 1-e 0+e],[0 0 1 1-e 0+e 0+e],c2);patch([0 0 1 1-e 0+e 0+e],[0 1 1 1-e 1-e 0+e],c3);plot([0 1 1 0 0],[0 0 1 1 0]);
  wires:
  "IW{1,1}(1,:)'"/1 -> dotprod1/1
  "pd{1,1}"/1 -> dotprod1/2, dotprod2/2, dotprod3/2, dotprod4/2, dotprod5/2, dotprod6/2, dotprod7/2, dotprod8/2, dotprod9/2, dotprod10/2
  dotprod1/1 -> Mux/1
  "IW{1,1}(2,:)'"/1 -> dotprod2/1
  dotprod2/1 -> Mux/2
  "IW{1,1}(3,:)'"/1 -> dotprod3/1
  dotprod3/1 -> Mux/3
  "IW{1,1}(4,:)'"/1 -> dotprod4/1
  dotprod4/1 -> Mux/4
  "IW{1,1}(5,:)'"/1 -> dotprod5/1
  dotprod5/1 -> Mux/5
  "IW{1,1}(6,:)'"/1 -> dotprod6/1
  dotprod6/1 -> Mux/6
  "IW{1,1}(7,:)'"/1 -> dotprod7/1
  dotprod7/1 -> Mux/7
  "IW{1,1}(8,:)'"/1 -> dotprod8/1
  dotprod8/1 -> Mux/8
  "IW{1,1}(9,:)'"/1 -> dotprod9/1
  dotprod9/1 -> Mux/9
  "IW{1,1}(10,:)'"/1 -> dotprod10/1
  dotprod10/1 -> Mux/10
  Mux/1 -> "iz{1,1}"/1

== system house_heat_model/NN Thermostat /NN predict/Function Fitting Neural Network1/Layer 2/Delays 1 ==
  "p{2}" : Inport  PortDimensions=10  SampleTime=10
      mask Display: e = 0.06;c1 = [120 230 180]/255;c2 = ([120 230 180]+0)/(256+128);c3 = ([120 230 180]+128)/(256+128);patch([0 1 1 0],[0 0 1 1],c1);patch([0 1 1 1-e 1-e 0+e],[0 0 1 1-e 0+e 0+e],c2);patch([0 0 1 1-e 0+e 0+e],[0 1 1 1-e 1-e 0+e],c3);plot([0 1 1 0 0],[0 0 1 1 0]);
  mux : Mux  Inputs=1
      mask Display: e = 0.06;c1 = [120 150 230]/255;c2 = ([120 150 230]+0)/383;c3 = ([120 150 230]+128)/383;patch([0 1 1 0],[0 0 1 1],c1);patch([0 1 1 1-e 1-e 0+e],[0 0 1 1-e 0+e 0+e],c2);patch([0 0 1 1-e 0+e 0+e],[0 1 1 1-e 1-e 0+e],c3);plot([0 1 1 0 0],[0 0 1 1 0]);disp('Mux')
  "pd{2,1}" : Outport
      mask Display: e = 0.06;c1 = [120 230 180]/255;c2 = ([120 230 180]+0)/(256+128);c3 = ([120 230 180]+128)/(256+128);patch([0 1 1 0],[0 0 1 1],c1);patch([0 1 1 1-e 1-e 0+e],[0 0 1 1-e 0+e 0+e],c2);patch([0 0 1 1-e 0+e 0+e],[0 1 1 1-e 1-e 0+e],c3);plot([0 1 1 0 0],[0 0 1 1 0]);
  wires:
  "p{2}"/1 -> mux/1
  mux/1 -> "pd{2,1}"/1

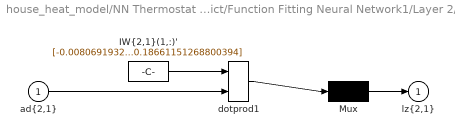
== system house_heat_model/NN Thermostat /NN predict/Function Fitting Neural Network1/Layer 2/LW{2,1} ==
  "ad{2,1}" : Inport  PortDimensions=10  SampleTime=10
      mask Display: e = 0.06;c1 = [120 230 180]/255;c2 = ([120 230 180]+0)/(256+128);c3 = ([120 230 180]+128)/(256+128);patch([0 1 1 0],[0 0 1 1],c1);patch([0 1 1 1-e 1-e 0+e],[0 0 1 1-e 0+e 0+e],c2);patch([0 0 1 1-e 0+e 0+e],[0 1 1 1-e 1-e 0+e],c3);plot([0 1 1 0 0],[0 0 1 1 0]);
  "IW{2,1}(1,:)'" : Constant  Value=[-0.0080691932473186331;0.2522757499612634;-0.29581554017668849;-0.3710360085072068;-0.010560420172121734;-0.054469232383010199;-0.11031493824886029;-0.17976599346782804;-0.24138539702046174;0.18661151268800394]
      mask Display: e = 0.06;c1 = [120 150 230]/255;c2 = ([120 150 230]+0)/383;c3 = ([120 150 230]+128)/383;patch([0 1 1 0],[0 0 1 1],c1);patch([0 1 1 1-e 1-e 0+e],[0 0 1 1-e 0+e 0+e],c2);patch([0 0 1 1-e 0+e 0+e],[0 1 1 1-e 1-e 0+e],c3);plot([0 1 1 0 0],[0 0 1 1 0]);disp('weights');
  Mux : Mux  Inputs=1
      mask Display: e = 0.06;c1 = [120 150 230]/255;c2 = ([120 150 230]+0)/383;c3 = ([120 150 230]+128)/383;patch([0 1 1 0],[0 0 1 1],c1);patch([0 1 1 1-e 1-e 0+e],[0 0 1 1-e 0+e 0+e],c2);patch([0 0 1 1-e 0+e 0+e],[0 1 1 1-e 1-e 0+e],c3);plot([0 1 1 0 0],[0 0 1 1 0]);disp('Mux');
  dotprod1 : neural/Weight Functions/dotprod
  "lz{2,1}" : Outport
      mask Display: e = 0.06;c1 = [120 230 180]/255;c2 = ([120 230 180]+0)/(256+128);c3 = ([120 230 180]+128)/(256+128);patch([0 1 1 0],[0 0 1 1],c1);patch([0 1 1 1-e 1-e 0+e],[0 0 1 1-e 0+e 0+e],c2);patch([0 0 1 1-e 0+e 0+e],[0 1 1 1-e 1-e 0+e],c3);plot([0 1 1 0 0],[0 0 1 1 0]);
  wires:
  "IW{2,1}(1,:)'"/1 -> dotprod1/1
  "ad{2,1}"/1 -> dotprod1/2
  dotprod1/1 -> Mux/1
  Mux/1 -> "lz{2,1}"/1

== matlab function house_heat_model/NN Thermostat /Predictor switch ==
  data: T input; T_1 input; T_2 input; y output; T_3 input; T_4 input
function y = fcn(T,T_1,T_2,T_3, T_4)
% overshoots

if (T>T_1) && (T_1>T_2) && (T_2>T_3) && (T_3>T_4)
    % rising temperature
    y=1;
else
    y=0;
end

== matlab function house_heat_model/Overshoots ==
  data: u input; y output; T input; T_1 input
function y = fcn(u,T,T_1)
% overshoots

if (u>0) && (T>T_1)
    % rising temperature
    y=u;
else
    y=0;
end

== matlab function house_heat_model/NN Thermostat /Relay ==
  data: y_1 input; dT input; T_upper input; y output; T_lower input
function y = fcn(y_1,dT,T_upper,T_lower)
% overshoots

if y_1==1 
    % rheating
    if (-dT>T_upper)
        y=0;
    else
        y=1;
    end
else
    % not heating
    if (dT>T_lower)
        y=1;
    else
        y=0;
    end
end
